simulink model "LOGIC_GATES"  (R2016a)
settings: Solver=VariableStepAuto  StartTime=0.0  StopTime=10  RelTol=1e-3  AbsTol=1e-3
settings Model: Creator=ec25227  LastModifiedBy=user
settings DataIOCC: LimitDataPoints=on  MaxDataPoints=10000
settings DebuggingCC: AllowSymbolicDim=off
settings ConfigComp: CovSFcnEnable=off
settings SimscapeCC: SimscapeLogType=all  SimscapeLogDataHistory=10000

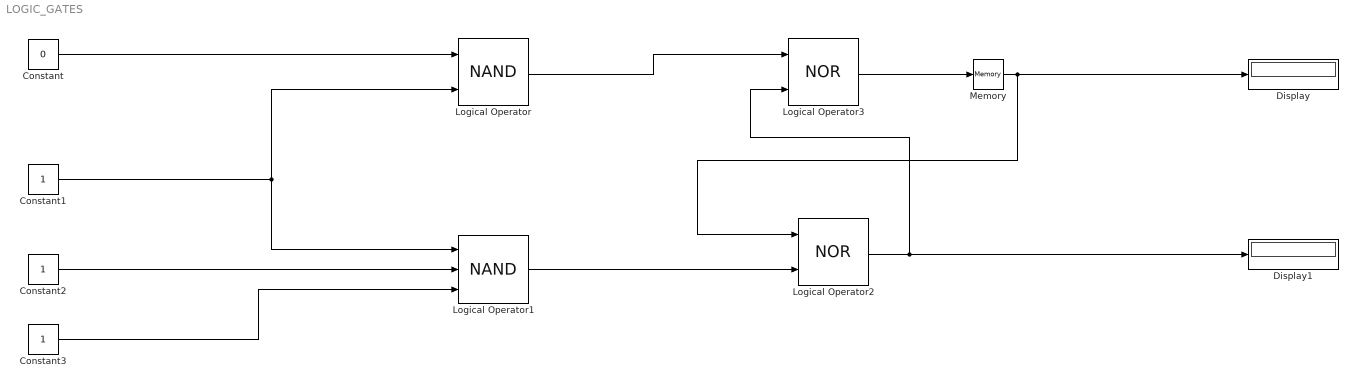
== system LOGIC_GATES ==
  Constant : Constant  Value=0
  Constant1 : Constant
  Constant2 : Constant
  Constant3 : Constant
  Display : Display
  Display1 : Display
  Logical Operator : Logic  Operator=NAND  AllPortsSameDT=off  OutDataTypeStr=boolean
  Logical Operator1 : Logic  Operator=NAND  Inputs=3  AllPortsSameDT=off  OutDataTypeStr=boolean
  Logical Operator2 : Logic  Operator=NOR  AllPortsSameDT=off  OutDataTypeStr=boolean
  Logical Operator3 : Logic  Operator=NOR  AllPortsSameDT=off  OutDataTypeStr=boolean
  Memory : Memory
  wires:
  Logical Operator/1 -> Logical Operator3/1
  Constant/1 -> Logical Operator/1
  Constant1/1 -> Logical Operator/2, Logical Operator1/1
  Constant2/1 -> Logical Operator1/2
  Logical Operator1/1 -> Logical Operator2/2
  Logical Operator3/1 -> Memory/1
  Memory/1 -> Display/1, Logical Operator2/1
  Logical Operator2/1 -> Display1/1, Logical Operator3/2
  Constant3/1 -> Logical Operator1/3
